simulink model "GENERADOR"  (R2018b)
settings: Solver=VariableStepAuto  StartTime=0.0  StopTime=20  RelTol=1e-3
settings Model: Creator=alvar  LastModifiedBy=alvar

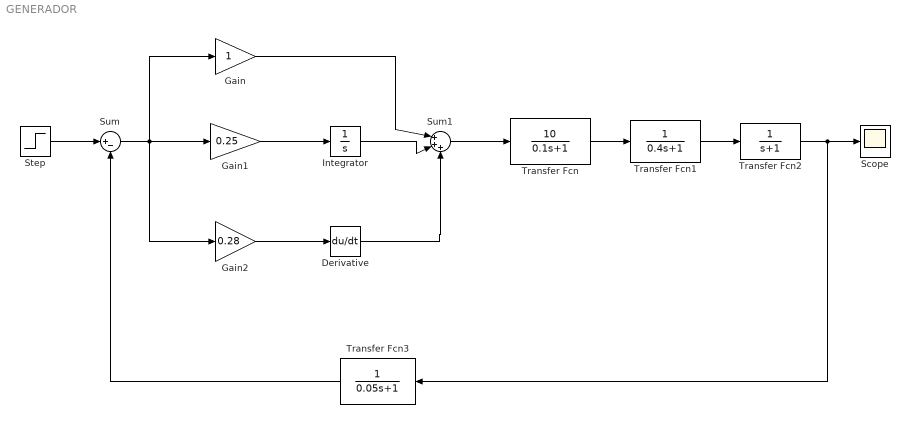
== system GENERADOR ==
  Derivative : Derivative
  Gain : Gain
  Gain1 : Gain  Gain=0.25
  Gain2 : Gain  Gain=0.28
  Integrator : Integrator
  Scope : Scope
  Step : Step  SampleTime=0
  Sum : Sum  Inputs=|+-
  Sum1 : Sum  Inputs=|+++
  Transfer Fcn : TransferFcn  Numerator=[10]  Denominator=[0.1 1]
  Transfer Fcn1 : TransferFcn  Denominator=[0.4 1]
  Transfer Fcn2 : TransferFcn  Denominator=[1 1]
  Transfer Fcn3 : TransferFcn  Denominator=[0.05 1]
  wires:
  Gain1/1 -> Integrator/1
  Gain2/1 -> Derivative/1
  Derivative/1 -> Sum1/3
  Integrator/1 -> Sum1/2
  Sum/1 -> Gain2/1, Gain/1, Gain1/1
  Step/1 -> Sum/1
  Sum1/1 -> Transfer Fcn/1
  Transfer Fcn/1 -> Transfer Fcn1/1
  Transfer Fcn1/1 -> Transfer Fcn2/1
  Transfer Fcn2/1 -> Transfer Fcn3/1, Scope/1
  Transfer Fcn3/1 -> Sum/2
  Gain/1 -> Sum1/1
